simulink model "dx_hand_model"  (R2017b)
settings: Solver=ode3  StartTime=0.0  StopTime=inf  FixedStep=0.01  RelTol=1e-3  EnableMultiTasking=on
InitFcn:
  | cutFreq = 0.1; % T
  | sampleTime = 0.01;
  | filt = tf(1,[cutFreq 1]);
  | filt = c2d(filt,sampleTime);
  | 
  | cutFreq2 = 1;
  | filt2 = tf(1,[cutFreq2 1]);
  | filt2 = c2d(filt2,sampleTime);
  | 
  | cutFreq3 = 0.3;
  | filt3 = tf(1,[cutFreq3 1]);
  | filt3 = c2d(filt3,sampleTime);
  | 
  | update_param = 2;
  | 
  | ampliFactor = 1.60;
  | ampliFactorMiddle = 2.00;
  | ampliFactorDistal = 1;
  | 
  | % Set Hand Address
  | % RightHandAddress = '10.100.39.144';
  | RightHandAddress = '10.24.4.91';
  | Verosim = '10.100.39.22'
  | LeftHandAddress = '10.100.39.22'
  | 
  | max_force = 24; % Newton
model workspace (MAT data in the model file):
  SL_ROS_VariableLengthArrays_MaxSizes : struct (value not decoded)
libraries: robotlib x136, simulink_extras x27, simulink x16, etargetslib x2, dspnetwork x2
(part 9 of 19)

== matlab function dx_hand_model/Thumb/Direct Kinematics/get H/MATLAB Function3 ==
  data: xI input; xH_sol output; yI input; zI input; xJ input; yJ input; zJ input; xD input; yD input; zD input; yH_sol output; zH_sol output; xold input; yold input; zold input
function [xH_sol,yH_sol,zH_sol] = findH_optimized(xI,yI,zI,xJ,yJ,zJ,xD,yD,zD,xold,yold,zold)
%FINDH_OPTIMIZED
%    [XH_SOL,YH_SOL,ZH_SOL] = FINDH_OPTIMIZED(XD,XI,XJ,YD,YI,YJ,ZD,ZI,ZJ)

%    This function was generated by the Symbolic Math Toolbox version 8.0.
%    08-Feb-2018 20:19:06

t2 = xD.^2;
t3 = xI.^2;
t4 = yD.^2;
t5 = yI.^2;
t6 = zD.^2;
t7 = zI.^2;
t8 = xD.*yI;
t9 = xJ.*yD;
t10 = xI.*yJ;
t645 = xI.*yD;
t646 = xD.*yJ;
t647 = xJ.*yI;
t11 = t8+t9+t10-t645-t646-t647;
t12 = 1.0./t11;
t13 = yJ.^2;
t14 = xJ.^2;
t15 = zJ.^2;
t16 = t3.^2;
t17 = t5.^2;
t88 = t2.*t7.*zI.*8.0;
t89 = t3.*t6.*zD.*4.0;
t90 = t6.*t14.*zD.*4.0;
t91 = t7.*t14.*zI.*4.0;
t92 = t4.*t7.*zI.*8.0;
t93 = t5.*t6.*zD.*4.0;
t94 = t6.*t13.*zD.*4.0;
t95 = t7.*t13.*zI.*4.0;
t96 = t3.*zD.*1.4916e4;
t97 = t16.*zD.*4.0;
t98 = t14.*zD.*1.4916e4;
t99 = t3.*zJ.*1.4916e4;
t100 = t14.*zI.*1.4916e4;
t101 = t16.*zJ.*4.0;
t102 = t5.*zD.*1.4916e4;
t103 = t17.*zD.*4.0;
t104 = t13.*zD.*1.4916e4;
t105 = t5.*zJ.*1.4916e4;
t106 = t13.*zI.*1.4916e4;
t107 = t17.*zJ.*4.0;
t108 = t3.*xD.*xI.*zD.*8.0;
t109 = t7.*xD.*xI.*zI.*4.0;
t110 = t3.*xD.*xI.*zI.*4.0;
t111 = t2.*xD.*xI.*zI.*4.0;
t112 = t7.*xD.*xJ.*zI.*1.2e1;
t113 = t3.*xD.*xI.*zJ.*1.2e1;
t114 = t6.*xI.*xJ.*zD.*8.0;
t115 = t2.*xD.*xI.*zJ.*4.0;
t116 = t2.*xD.*xJ.*zI.*4.0;
t117 = t3.*xI.*xJ.*zD.*8.0;
t118 = t2.*xD.*xJ.*zJ.*4.0;
t119 = t7.*xI.*xJ.*zI.*4.0;
t120 = t3.*xI.*xJ.*zI.*4.0;
t121 = t3.*xI.*xJ.*zJ.*4.0;
t122 = t5.*yD.*yI.*zD.*8.0;
t123 = t7.*yD.*yI.*zI.*4.0;
t124 = t5.*yD.*yI.*zI.*4.0;
t125 = t4.*yD.*yI.*zI.*4.0;
t126 = t7.*yD.*yJ.*zI.*1.2e1;
t127 = t5.*yD.*yI.*zJ.*1.2e1;
t128 = t6.*yI.*yJ.*zD.*8.0;
t129 = t4.*yD.*yI.*zJ.*4.0;
t130 = t4.*yD.*yJ.*zI.*4.0;
t131 = t5.*yI.*yJ.*zD.*8.0;
t132 = t4.*yD.*yJ.*zJ.*4.0;
t133 = t7.*yI.*yJ.*zI.*4.0;
t134 = t5.*yI.*yJ.*zI.*4.0;
t135 = t5.*yI.*yJ.*zJ.*4.0;
t136 = t2.*t3.*zD.*4.0;
t137 = t2.*t14.*zD.*4.0;
t138 = t2.*t3.*zI.*8.0;
t139 = t2.*t3.*zJ.*1.2e1;
t140 = t2.*t14.*zI.*4.0;
t141 = t3.*t14.*zD.*4.0;
t142 = t3.*t14.*zI.*4.0;
t143 = t2.*t5.*zD.*4.0;
t144 = t3.*t4.*zD.*4.0;
t145 = t2.*t13.*zD.*4.0;
t146 = t4.*t14.*zD.*4.0;
t147 = t2.*t5.*zI.*8.0;
t148 = t3.*t4.*zI.*8.0;
t149 = t3.*t5.*zD.*8.0;
t150 = t2.*t5.*zJ.*4.0;
t151 = t2.*t13.*zI.*4.0;
t152 = t3.*t4.*zJ.*4.0;
t153 = t3.*t13.*zD.*4.0;
t154 = t4.*t14.*zI.*4.0;
t155 = t5.*t14.*zD.*4.0;
t156 = t3.*t5.*zJ.*8.0;
t157 = t3.*t13.*zI.*4.0;
t158 = t5.*t14.*zI.*4.0;
t159 = t4.*t5.*zD.*4.0;
t160 = t4.*t13.*zD.*4.0;
t161 = t3.*t7.*zD.*4.0;
t162 = t4.*t5.*zI.*8.0;
t163 = t2.*t15.*zI.*8.0;
t164 = t2.*t7.*zJ.*1.6e1;
t165 = t3.*t6.*zJ.*4.0;
t166 = t7.*t14.*zD.*4.0;
t167 = t6.*t14.*zI.*4.0;
t168 = t4.*t5.*zJ.*1.2e1;
t169 = t4.*t13.*zI.*4.0;
t170 = t5.*t13.*zD.*4.0;
t171 = t3.*t15.*zI.*8.0;
t172 = t3.*t7.*zJ.*4.0;
t173 = t5.*t13.*zI.*4.0;
t174 = t5.*t7.*zD.*4.0;
t175 = t4.*t15.*zI.*8.0;
t176 = t4.*t7.*zJ.*1.6e1;
t177 = t5.*t6.*zJ.*4.0;
t178 = t7.*t13.*zD.*4.0;
t179 = t6.*t13.*zI.*4.0;
t180 = t5.*t15.*zI.*8.0;
t181 = t5.*t7.*zJ.*4.0;
t182 = xD.*xI.*zI.*1.4916e4;
t183 = xD.*xI.*zJ.*1.4916e4;
t184 = xD.*xJ.*zI.*1.4916e4;
t185 = xI.*xJ.*zD.*2.9832e4;
t186 = xD.*xJ.*zJ.*1.4916e4;
t187 = xI.*xJ.*zI.*1.4916e4;
t188 = xI.*xJ.*zJ.*1.4916e4;
t189 = yD.*yI.*zI.*1.4916e4;
t190 = yD.*yI.*zJ.*1.4916e4;
t191 = yD.*yJ.*zI.*1.4916e4;
t192 = yI.*yJ.*zD.*2.9832e4;
t193 = yD.*yJ.*zJ.*1.4916e4;
t194 = yI.*yJ.*zI.*1.4916e4;
t195 = yI.*yJ.*zJ.*1.4916e4;
t196 = t14.*xD.*xI.*zD.*8.0;
t197 = t3.*xD.*xJ.*zD.*1.6e1;
t198 = t2.*xI.*xJ.*zD.*8.0;
t199 = t14.*xD.*xI.*zI.*8.0;
t200 = t3.*xD.*xJ.*zI.*4.0;
t201 = t2.*xI.*xJ.*zI.*4.0;
t202 = t3.*xD.*xJ.*zJ.*1.2e1;
t203 = t2.*xI.*xJ.*zJ.*1.2e1;
t204 = t4.*xD.*xI.*zI.*4.0;
t205 = t5.*xD.*xI.*zD.*8.0;
t206 = t4.*xD.*xI.*zJ.*4.0;
t207 = t13.*xD.*xI.*zD.*8.0;
t208 = t4.*xD.*xJ.*zI.*4.0;
t209 = t4.*xI.*xJ.*zD.*8.0;
t210 = t4.*xD.*xJ.*zJ.*4.0;
t211 = t5.*xD.*xI.*zI.*4.0;
t212 = t5.*xD.*xI.*zJ.*1.2e1;
t213 = t13.*xD.*xI.*zI.*8.0;
t214 = t5.*xD.*xJ.*zI.*1.2e1;
t215 = t4.*xI.*xJ.*zI.*1.2e1;
t216 = t5.*xI.*xJ.*zD.*8.0;
t217 = t5.*xD.*xJ.*zJ.*4.0;
t218 = t4.*xI.*xJ.*zJ.*4.0;
t219 = t5.*xI.*xJ.*zI.*4.0;
t220 = t5.*xI.*xJ.*zJ.*4.0;
t221 = t7.*xD.*xI.*zD.*8.0;
t222 = t6.*xD.*xI.*zI.*4.0;
t223 = t2.*yD.*yI.*zI.*4.0;
t224 = t3.*yD.*yI.*zD.*8.0;
t225 = t6.*xD.*xI.*zJ.*4.0;
t226 = t7.*xD.*xJ.*zD.*8.0;
t227 = t6.*xD.*xJ.*zI.*4.0;
t228 = t2.*yD.*yI.*zJ.*4.0;
t229 = t2.*yD.*yJ.*zI.*4.0;
t230 = t2.*yI.*yJ.*zD.*8.0;
t231 = t14.*yD.*yI.*zD.*8.0;
t232 = t6.*xD.*xJ.*zJ.*4.0;
t233 = t2.*yD.*yJ.*zJ.*4.0;
t234 = t3.*yD.*yI.*zI.*4.0;
t235 = t15.*xD.*xI.*zI.*1.6e1;
t236 = t7.*xD.*xI.*zJ.*2.0e1;
t237 = t6.*xI.*xJ.*zI.*4.0;
t238 = t2.*yI.*yJ.*zI.*1.2e1;
t239 = t3.*yD.*yI.*zJ.*1.2e1;
t240 = t3.*yD.*yJ.*zI.*1.2e1;
t241 = t3.*yI.*yJ.*zD.*8.0;
t242 = t14.*yD.*yI.*zI.*8.0;
t243 = t7.*xD.*xJ.*zJ.*1.2e1;
t244 = t6.*xI.*xJ.*zJ.*4.0;
t245 = t2.*yI.*yJ.*zJ.*4.0;
t246 = t3.*yD.*yJ.*zJ.*4.0;
t247 = t3.*yI.*yJ.*zI.*4.0;
t248 = t7.*xI.*xJ.*zJ.*1.2e1;
t249 = t3.*yI.*yJ.*zJ.*4.0;
t250 = t13.*yD.*yI.*zD.*8.0;
t251 = t5.*yD.*yJ.*zD.*1.6e1;
t252 = t4.*yI.*yJ.*zD.*8.0;
t253 = t13.*yD.*yI.*zI.*8.0;
t254 = t5.*yD.*yJ.*zI.*4.0;
t255 = t4.*yI.*yJ.*zI.*4.0;
t256 = t5.*yD.*yJ.*zJ.*1.2e1;
t257 = t4.*yI.*yJ.*zJ.*1.2e1;
t258 = t7.*yD.*yI.*zD.*8.0;
t259 = t6.*yD.*yI.*zI.*4.0;
t260 = t6.*yD.*yI.*zJ.*4.0;
t261 = t7.*yD.*yJ.*zD.*8.0;
t262 = t6.*yD.*yJ.*zI.*4.0;
t263 = t6.*yD.*yJ.*zJ.*4.0;
t264 = t15.*yD.*yI.*zI.*1.6e1;
t265 = t7.*yD.*yI.*zJ.*2.0e1;
t266 = t6.*yI.*yJ.*zI.*4.0;
t267 = t3.*zD.*zI.*zJ.*8.0;
t268 = t7.*yD.*yJ.*zJ.*1.2e1;
t269 = t6.*yI.*yJ.*zJ.*4.0;
t270 = t7.*yI.*yJ.*zJ.*1.2e1;
t271 = t5.*zD.*zI.*zJ.*8.0;
t272 = xD.*xI.*yD.*yI.*zJ.*1.6e1;
t273 = xD.*xI.*yD.*yJ.*zI.*8.0;
t274 = xD.*xI.*yI.*yJ.*zD.*1.6e1;
t275 = xD.*xJ.*yD.*yI.*zI.*8.0;
t276 = xI.*xJ.*yD.*yI.*zD.*1.6e1;
t277 = xD.*xI.*yD.*yJ.*zJ.*8.0;
t278 = xD.*xJ.*yD.*yI.*zJ.*8.0;
t279 = xD.*xJ.*yD.*yJ.*zI.*1.6e1;
t280 = xD.*xI.*yI.*yJ.*zI.*8.0;
t281 = xI.*xJ.*yD.*yI.*zI.*8.0;
t282 = xD.*xI.*yI.*yJ.*zJ.*8.0;
t283 = xD.*xJ.*yI.*yJ.*zI.*1.6e1;
t284 = xI.*xJ.*yD.*yI.*zJ.*8.0;
t285 = xI.*xJ.*yD.*yJ.*zI.*1.6e1;
t286 = xI.*xJ.*yI.*yJ.*zI.*1.6e1;
t287 = xD.*xI.*zD.*zI.*zJ.*8.0;
t288 = xD.*xJ.*zD.*zI.*zJ.*8.0;
t289 = xI.*xJ.*zD.*zI.*zJ.*8.0;
t290 = yD.*yI.*zD.*zI.*zJ.*8.0;
t291 = yD.*yJ.*zD.*zI.*zJ.*8.0;
t292 = yI.*yJ.*zD.*zI.*zJ.*8.0;
t18 = t88+t89+t90+t91+t92+t93+t94+t95-t96+t97-t98+t99+t100-t101-t102+t103-t104+t105+t106-t107-t108-t109-t110-t111-t112+t113-t114+t115+t116-t117-t118+t119+t120+t121-t122-t123-t124-t125-t126+t127-t128+t129+t130-t131-t132+t133+t134+t135+t136+t137+t138-t139-t140+t141-t142+t143+t144+t145+t146+t147+t148+t149-t150+t151-t152+t153+t154+t155-t156+t157+t158+t159+t160+t161+t162+t163-t164-t165-t166-t167-t168-t169+t170+t171-t172-t173+t174+t175-t176-t177-t178-t179+t180-t181+t182-t183-t184+t185+t186-t187-t188+t189-t190-t191+t192+t193-t194-t195-t196+t197-t198+t199-t200-t201-t202+t203-t204-t205+t206-t207+t208-t209-t210-t211+t212-t213-t214-t215-t216-t217+t218+t219+t220-t221-t222-t223-t224+t225+t226+t227+t228+t229-t230-t231-t232-t233-t234-t235+t236+t237-t238+t239-t240-t241-t242+t243+t244+t245-t246+t247-t248+t249-t250+t251-t252+t253-t254-t255-t256+t257-t258-t259+t260+t261+t262-t263-t264+t265+t266-t267+t268+t269-t270-t271-t272+t273+t274+t275+t276+t277+t278-t279+t280+t281-t282+t283-t284+t285-t286+t287-t288+t289+t290-t291+t292;
t19 = t2.*t5.*4.0;
t20 = t3.*t4.*4.0;
t21 = t2.*t13.*4.0;
t22 = t4.*t14.*4.0;
t23 = t3.*t13.*4.0;
t24 = t5.*t14.*4.0;
t25 = t2.*t7.*4.0;
t26 = t3.*t6.*4.0;
t27 = t2.*t15.*4.0;
t28 = t6.*t14.*4.0;
t29 = t3.*t15.*4.0;
t30 = t7.*t14.*4.0;
t31 = t4.*t7.*4.0;
t32 = t5.*t6.*4.0;
t33 = t4.*t15.*4.0;
t34 = t6.*t13.*4.0;
t35 = t5.*t15.*4.0;
t36 = t7.*t13.*4.0;
t37 = xD.*xI.*yD.*yJ.*8.0;
t38 = xD.*xJ.*yD.*yI.*8.0;
t39 = xD.*xI.*yI.*yJ.*8.0;
t40 = xI.*xJ.*yD.*yI.*8.0;
t41 = xD.*xJ.*yI.*yJ.*8.0;
t42 = xI.*xJ.*yD.*yJ.*8.0;
t43 = xD.*xI.*zD.*zJ.*8.0;
t44 = xD.*xJ.*zD.*zI.*8.0;
t45 = xD.*xI.*zI.*zJ.*8.0;
t46 = xI.*xJ.*zD.*zI.*8.0;
t47 = xD.*xJ.*zI.*zJ.*8.0;
t48 = xI.*xJ.*zD.*zJ.*8.0;
t49 = yD.*yI.*zD.*zJ.*8.0;
t50 = yD.*yJ.*zD.*zI.*8.0;
t51 = yD.*yI.*zI.*zJ.*8.0;
t52 = yI.*yJ.*zD.*zI.*8.0;
t53 = yD.*yJ.*zI.*zJ.*8.0;
t54 = yI.*yJ.*zD.*zJ.*8.0;
t60 = t13.*xD.*xI.*8.0;
t61 = t5.*xD.*xJ.*8.0;
t62 = t4.*xI.*xJ.*8.0;
t63 = t15.*xD.*xI.*8.0;
t64 = t7.*xD.*xJ.*8.0;
t65 = t6.*xI.*xJ.*8.0;
t66 = t2.*yI.*yJ.*8.0;
t67 = t3.*yD.*yJ.*8.0;
t68 = t14.*yD.*yI.*8.0;
t69 = t15.*yD.*yI.*8.0;
t70 = t7.*yD.*yJ.*8.0;
t71 = t6.*yI.*yJ.*8.0;
t72 = t2.*zI.*zJ.*8.0;
t73 = t3.*zD.*zJ.*8.0;
t74 = t14.*zD.*zI.*8.0;
t75 = t4.*zI.*zJ.*8.0;
t76 = t5.*zD.*zJ.*8.0;
t77 = t13.*zD.*zI.*8.0;
t78 = xD.*xI.*yD.*yI.*8.0;
t79 = xD.*xJ.*yD.*yJ.*8.0;
t80 = xI.*xJ.*yI.*yJ.*8.0;
t81 = xD.*xI.*zD.*zI.*8.0;
t82 = xD.*xJ.*zD.*zJ.*8.0;
t83 = xI.*xJ.*zI.*zJ.*8.0;
t84 = yD.*yI.*zD.*zI.*8.0;
t85 = yD.*yJ.*zD.*zJ.*8.0;
t86 = yI.*yJ.*zI.*zJ.*8.0;
t55 = t19+t20+t21+t22+t23+t24+t25+t26+t27+t28+t29+t30+t31+t32+t33+t34+t35+t36+t37+t38+t39+t40+t41+t42+t43+t44+t45+t46+t47+t48+t49+t50+t51+t52+t53+t54-t60-t61-t62-t63-t64-t65-t66-t67-t68-t69-t70-t71-t72-t73-t74-t75-t76-t77-t78-t79-t80-t81-t82-t83-t84-t85-t86;
t56 = t2.^2;
t57 = t4.^2;
t58 = t6.^2;
t59 = t7.^2;
t87 = 1.0./t55.^2;
t293 = t18.^2;
t294 = t87.*t293.*(1.0./4.0);
t295 = 1.0./t55;
t296 = t2.*t16.*6.0;
t297 = t3.*t56;
t298 = t14.*t56;
t299 = t14.*t16;
t300 = t2.*t17.*2.0;
t301 = t5.*t56;
t302 = t3.*t57;
t303 = t4.*t16.*2.0;
t304 = t13.*t56;
t305 = t14.*t57;
t306 = t3.*t17.*3.0;
t307 = t5.*t16.*3.0;
t308 = t13.*t16;
t309 = t14.*t17;
t310 = t2.*t59.*4.0;
t311 = t3.*t58;
t312 = t6.*t16.*2.0;
t313 = t4.*t17.*6.0;
t314 = t5.*t57;
t315 = t14.*t58;
t316 = t13.*t57;
t317 = t3.*t59;
t318 = t7.*t16.*2.0;
t319 = t7.*t14.*7.458e3;
t320 = t14.*t59;
t321 = t13.*t17;
t322 = t4.*t59.*4.0;
t323 = t5.*t58;
t324 = t6.*t17.*2.0;
t325 = t13.*t58;
t326 = t5.*t59;
t327 = t7.*t17.*2.0;
t328 = t7.*t13.*7.458e3;
t329 = t13.*t59;
t330 = t3.*xD.*xI.*1.4916e4;
t331 = t3.*xI.*xJ.*1.4916e4;
t332 = t5.*yD.*yI.*1.4916e4;
t333 = t5.*yI.*yJ.*1.4916e4;
t334 = t3.*1.3905441e7;
t335 = t14.*1.3905441e7;
t336 = t5.*1.3905441e7;
t337 = t13.*1.3905441e7;
t338 = t14.*xD.*xI.*1.4916e4;
t339 = t2.*xI.*xJ.*1.4916e4;
t340 = t16.*xD.*xJ.*8.0;
t341 = t5.*xD.*xI.*1.4916e4;
t342 = t13.*xD.*xI.*2.7716e4;
t343 = t5.*xD.*xJ.*1.28e4;
t344 = t4.*xI.*xJ.*2.7716e4;
t345 = t5.*xI.*xJ.*1.4916e4;
t346 = t7.*xD.*xI.*1.4916e4;
t347 = t3.*yD.*yI.*1.4916e4;
t348 = t6.*xI.*xJ.*1.4916e4;
t349 = t2.*yI.*yJ.*2.7716e4;
t350 = t3.*yD.*yJ.*1.28e4;
t351 = t14.*yD.*yI.*2.7716e4;
t352 = t3.*yI.*yJ.*1.4916e4;
t353 = t59.*xI.*xJ.*2.0;
t354 = t13.*yD.*yI.*1.4916e4;
t355 = t4.*yI.*yJ.*1.4916e4;
t356 = t17.*yD.*yJ.*8.0;
t357 = t7.*yD.*yI.*1.4916e4;
t358 = t6.*yI.*yJ.*1.4916e4;
t359 = t3.*zI.*zJ.*1.4916e4;
t360 = t59.*yI.*yJ.*2.0;
t361 = t5.*zI.*zJ.*1.4916e4;
t362 = t2.*t3.*xD.*xJ.*8.0;
t363 = t2.*t7.*xD.*xJ.*4.0;
t364 = t4.*t5.*yD.*yJ.*8.0;
t365 = t4.*t7.*yD.*yJ.*4.0;
t366 = t2.*t3.*t14.*6.0;
t367 = t2.*t3.*t4.*2.0;
t368 = t2.*t4.*t14.*2.0;
t369 = t2.*t3.*t5.*8.0;
t370 = t2.*t3.*t13.*6.0;
t371 = t2.*t5.*t14.*2.0;
t372 = t3.*t4.*t14.*2.0;
t373 = t3.*t5.*t14.*2.0;
t374 = t2.*t3.*t6.*2.0;
t375 = t2.*t4.*t5.*2.0;
t376 = t2.*t6.*t14.*2.0;
t377 = t2.*t4.*t13.*2.0;
t378 = t2.*t3.*t7.*1.0e1;
t379 = t3.*t4.*t5.*8.0;
t380 = t2.*t5.*t13.*2.0;
t381 = t3.*t6.*t14.*2.0;
t382 = t3.*t4.*t13.*2.0;
t383 = t4.*t5.*t14.*6.0;
t384 = t3.*t5.*t13.*2.0;
t385 = t2.*t5.*t6.*2.0;
t386 = t3.*t4.*t6.*2.0;
t387 = t2.*t6.*t13.*2.0;
t388 = t4.*t6.*t14.*2.0;
t389 = t2.*t5.*t7.*6.0;
t390 = t3.*t4.*t7.*6.0;
t391 = t3.*t5.*t6.*4.0;
t392 = t2.*t7.*t13.*2.0;
t393 = t3.*t6.*t13.*2.0;
t394 = t4.*t7.*t14.*2.0;
t395 = t5.*t6.*t14.*2.0;
t396 = t4.*t5.*t13.*6.0;
t397 = t3.*t5.*t7.*4.0;
t398 = t3.*t7.*t13.*2.0;
t399 = t5.*t7.*t14.*2.0;
t400 = t4.*t5.*t6.*2.0;
t401 = t4.*t6.*t13.*2.0;
t402 = t3.*t6.*t7.*2.0;
t403 = t4.*t5.*t7.*1.0e1;
t404 = t2.*t7.*t15.*4.0;
t405 = t5.*t6.*t13.*2.0;
t406 = t3.*t7.*t15.*4.0;
t407 = t5.*t6.*t7.*2.0;
t408 = t4.*t7.*t15.*4.0;
t409 = t5.*t7.*t15.*4.0;
t410 = t3.*t4.*xD.*xJ.*8.0;
t411 = t3.*t5.*xD.*xJ.*8.0;
t412 = t3.*t6.*xD.*xJ.*8.0;
t413 = t7.*t14.*xD.*xI.*4.0;
t414 = t3.*t7.*xD.*xJ.*4.0;
t415 = t4.*t7.*xD.*xJ.*4.0;
t416 = t2.*t5.*yD.*yJ.*8.0;
t417 = t3.*t5.*yD.*yJ.*8.0;
t418 = t6.*t7.*xD.*xJ.*4.0;
t419 = t2.*t7.*yD.*yJ.*4.0;
t420 = t5.*t6.*yD.*yJ.*8.0;
t421 = t7.*t13.*yD.*yI.*4.0;
t422 = t5.*t7.*yD.*yJ.*4.0;
t423 = t6.*t7.*yD.*yJ.*4.0;
t424 = xD.*xI.*yD.*yI.*1.28e4;
t425 = xD.*xJ.*yD.*yJ.*1.28e4;
t426 = xI.*xJ.*yI.*yJ.*1.28e4;
t427 = xD.*xJ.*zI.*zJ.*1.4916e4;
t428 = yD.*yJ.*zI.*zJ.*1.4916e4;
t429 = t5.*xD.*xI.*yD.*yI.*8.0;
t430 = t3.*xD.*xI.*yD.*yI.*8.0;
t431 = t5.*xD.*xI.*yI.*yJ.*8.0;
t432 = t3.*xD.*xI.*yI.*yJ.*8.0;
t433 = t5.*xI.*xJ.*yD.*yI.*8.0;
t434 = t4.*xI.*xJ.*yD.*yI.*8.0;
t435 = t2.*xD.*xI.*yI.*yJ.*8.0;
t436 = t3.*xI.*xJ.*yD.*yI.*8.0;
t437 = t7.*xD.*xI.*zI.*zJ.*1.2e1;
t438 = t3.*xD.*xI.*zI.*zJ.*1.2e1;
t439 = t2.*xD.*xI.*zI.*zJ.*4.0;
t440 = t7.*xD.*xJ.*zI.*zJ.*4.0;
t441 = t3.*xI.*xJ.*zI.*zJ.*4.0;
t442 = t7.*yD.*yI.*zI.*zJ.*1.2e1;
t443 = t5.*yD.*yI.*zI.*zJ.*1.2e1;
t444 = t4.*yD.*yI.*zI.*zJ.*4.0;
t445 = t7.*yD.*yJ.*zI.*zJ.*4.0;
t446 = t5.*yI.*yJ.*zI.*zJ.*4.0;
t447 = t14.*xD.*xI.*yD.*yI.*8.0;
t448 = t2.*xI.*xJ.*yD.*yI.*8.0;
t449 = t13.*xD.*xI.*yD.*yI.*8.0;
t450 = t4.*xD.*xI.*yI.*yJ.*8.0;
t451 = t7.*xD.*xI.*yD.*yI.*8.0;
t452 = t6.*xD.*xI.*yI.*yJ.*8.0;
t453 = t6.*xI.*xJ.*yD.*yI.*8.0;
t454 = t7.*xD.*xI.*yI.*yJ.*8.0;
t455 = t7.*xI.*xJ.*yD.*yI.*8.0;
t456 = t7.*xD.*xJ.*yI.*yJ.*8.0;
t457 = t7.*xI.*xJ.*yD.*yJ.*8.0;
t458 = t2.*xI.*xJ.*zI.*zJ.*1.2e1;
t459 = t4.*xD.*xI.*zI.*zJ.*4.0;
t460 = t5.*xD.*xI.*zI.*zJ.*1.2e1;
t461 = t4.*xI.*xJ.*zI.*zJ.*4.0;
t462 = t5.*xI.*xJ.*zI.*zJ.*4.0;
t463 = t6.*xD.*xI.*zI.*zJ.*4.0;
t464 = t2.*yD.*yI.*zI.*zJ.*4.0;
t465 = t3.*yD.*yI.*zI.*zJ.*1.2e1;
t466 = t6.*xI.*xJ.*zI.*zJ.*4.0;
t467 = t2.*yI.*yJ.*zI.*zJ.*4.0;
t468 = t3.*yI.*yJ.*zI.*zJ.*4.0;
t469 = t4.*yI.*yJ.*zI.*zJ.*1.2e1;
t470 = t6.*yD.*yI.*zI.*zJ.*4.0;
t471 = t6.*yI.*yJ.*zI.*zJ.*4.0;
t472 = xD.*xI.*yD.*yJ.*zI.*zJ.*8.0;
t473 = xD.*xJ.*yD.*yI.*zI.*zJ.*8.0;
t477 = t2.*t3.*7.458e3;
t478 = t2.*t3.*xD.*xI.*4.0;
t479 = t2.*t14.*7.458e3;
t480 = t3.*t14.*7.458e3;
t481 = t2.*t5.*1.3858e4;
t482 = t3.*t4.*1.3858e4;
t483 = t2.*t13.*1.3858e4;
t484 = t4.*t14.*1.3858e4;
t485 = t3.*t5.*1.4916e4;
t486 = t3.*t13.*1.3858e4;
t487 = t5.*t14.*1.3858e4;
t488 = t3.*t6.*7.458e3;
t489 = t4.*t5.*7.458e3;
t490 = t4.*t5.*yD.*yI.*4.0;
t491 = t6.*t14.*7.458e3;
t492 = t4.*t13.*7.458e3;
t493 = t3.*t7.*7.458e3;
t494 = t5.*t13.*7.458e3;
t495 = t5.*t6.*7.458e3;
t496 = t6.*t13.*7.458e3;
t497 = t5.*t7.*7.458e3;
t498 = xI.*xJ.*2.7810882e7;
t499 = yI.*yJ.*2.7810882e7;
t500 = t16.*xD.*xI.*4.0;
t501 = t16.*xI.*xJ.*2.0;
t502 = t17.*yD.*yI.*4.0;
t503 = t17.*yI.*yJ.*2.0;
t504 = t16.*7.458e3;
t505 = t17.*7.458e3;
t506 = t3.*xD.*xJ.*2.9832e4;
t507 = t56.*xI.*xJ.*2.0;
t508 = t17.*xD.*xI.*4.0;
t509 = t57.*xI.*xJ.*2.0;
t510 = t17.*xI.*xJ.*2.0;
t511 = t59.*xD.*xI.*4.0;
t512 = t16.*yD.*yI.*4.0;
t513 = t7.*xD.*xJ.*1.4916e4;
t514 = t59.*xD.*xJ.*4.0;
t515 = t58.*xI.*xJ.*2.0;
t516 = t56.*yI.*yJ.*2.0;
t517 = t16.*yI.*yJ.*2.0;
t518 = t5.*yD.*yJ.*2.9832e4;
t519 = t57.*yI.*yJ.*2.0;
t520 = t59.*yD.*yI.*4.0;
t521 = t7.*yD.*yJ.*1.4916e4;
t522 = t59.*yD.*yJ.*4.0;
t523 = t58.*yI.*yJ.*2.0;
t524 = t16.*zI.*zJ.*4.0;
t525 = t17.*zI.*zJ.*4.0;
t526 = t3.*t14.*xD.*xI.*4.0;
t527 = t2.*t3.*xI.*xJ.*1.2e1;
t528 = t2.*t14.*xD.*xI.*4.0;
t529 = t3.*t4.*xD.*xI.*4.0;
t530 = t3.*t5.*xD.*xI.*8.0;
t531 = t2.*t5.*xD.*xI.*4.0;
t532 = t3.*t13.*xD.*xI.*4.0;
t533 = t2.*t13.*xD.*xI.*4.0;
t534 = t3.*t4.*xI.*xJ.*4.0;
t535 = t3.*t5.*xI.*xJ.*4.0;
t536 = t3.*t6.*xD.*xI.*4.0;
t537 = t2.*t5.*yD.*yI.*4.0;
t538 = t3.*t7.*xD.*xI.*8.0;
t539 = t2.*t7.*xD.*xI.*4.0;
t540 = t3.*t5.*yD.*yI.*8.0;
t541 = t3.*t4.*yD.*yI.*4.0;
t542 = t2.*t5.*yI.*yJ.*4.0;
t543 = t3.*t6.*xI.*xJ.*4.0;
t544 = t5.*t14.*yD.*yI.*4.0;
t545 = t4.*t14.*yD.*yI.*4.0;
t546 = t3.*t5.*yI.*yJ.*4.0;
t547 = t5.*t13.*yD.*yI.*4.0;
t548 = t4.*t5.*yI.*yJ.*1.2e1;
t549 = t4.*t13.*yD.*yI.*4.0;
t550 = t5.*t6.*yD.*yI.*4.0;
t551 = t5.*t7.*yD.*yI.*8.0;
t552 = t4.*t7.*yD.*yI.*4.0;
t553 = t2.*t7.*zI.*zJ.*8.0;
t554 = t5.*t6.*yI.*yJ.*4.0;
t555 = t3.*t7.*zI.*zJ.*4.0;
t556 = t4.*t7.*zI.*zJ.*8.0;
t557 = t5.*t7.*zI.*zJ.*4.0;
t558 = t2.*t7.*t14.*2.0;
t559 = t3.*t7.*t14.*2.0;
t560 = t6.*t7.*t14.*2.0;
t561 = t4.*t7.*t13.*2.0;
t562 = t5.*t7.*t13.*2.0;
t563 = t6.*t7.*t13.*2.0;
t564 = t4.*t14.*xD.*xI.*4.0;
t565 = t2.*t4.*xI.*xJ.*4.0;
t566 = t5.*t14.*xD.*xI.*4.0;
t567 = t2.*t5.*xI.*xJ.*4.0;
t568 = t4.*t5.*xD.*xI.*4.0;
t569 = t2.*t3.*yD.*yI.*4.0;
t570 = t6.*t14.*xD.*xI.*4.0;
t571 = t4.*t13.*xD.*xI.*4.0;
t572 = t2.*t6.*xI.*xJ.*4.0;
t573 = t2.*t14.*yD.*yI.*4.0;
t574 = t5.*t13.*xD.*xI.*4.0;
t575 = t4.*t5.*xI.*xJ.*1.2e1;
t576 = t2.*t7.*xI.*xJ.*8.0;
t577 = t2.*t3.*yI.*yJ.*1.2e1;
t578 = t3.*t14.*yD.*yI.*4.0;
t579 = t4.*t7.*xD.*xI.*4.0;
t580 = t5.*t6.*xD.*xI.*4.0;
t581 = t6.*t13.*xD.*xI.*4.0;
t582 = t4.*t6.*xI.*xJ.*4.0;
t583 = t2.*t13.*yD.*yI.*4.0;
t584 = t2.*t4.*yI.*yJ.*4.0;
t585 = t5.*t7.*xD.*xI.*8.0;
t586 = t7.*t13.*xD.*xI.*4.0;
t587 = t5.*t7.*xD.*xJ.*4.0;
t588 = t4.*t7.*xI.*xJ.*8.0;
t589 = t5.*t6.*xI.*xJ.*4.0;
t590 = t3.*t13.*yD.*yI.*4.0;
t591 = t3.*t4.*yI.*yJ.*4.0;
t592 = t6.*t7.*xD.*xI.*4.0;
t593 = t2.*t7.*yD.*yI.*4.0;
t594 = t3.*t6.*yD.*yI.*4.0;
t595 = t2.*t6.*yI.*yJ.*4.0;
t596 = t6.*t14.*yD.*yI.*4.0;
t597 = t3.*t7.*yD.*yI.*8.0;
t598 = t7.*t15.*xD.*xI.*8.0;
t599 = t2.*t7.*yI.*yJ.*8.0;
t600 = t2.*t3.*zI.*zJ.*1.2e1;
t601 = t3.*t7.*yD.*yJ.*4.0;
t602 = t3.*t6.*yI.*yJ.*4.0;
t603 = t7.*t14.*yD.*yI.*4.0;
t604 = t6.*t13.*yD.*yI.*4.0;
t605 = t4.*t6.*yI.*yJ.*4.0;
t606 = t2.*t5.*zI.*zJ.*4.0;
t607 = t3.*t4.*zI.*zJ.*4.0;
t608 = t4.*t7.*yI.*yJ.*8.0;
t609 = t3.*t5.*zI.*zJ.*8.0;
t610 = t6.*t7.*yD.*yI.*4.0;
t611 = t7.*t15.*yD.*yI.*8.0;
t612 = t3.*t6.*zI.*zJ.*4.0;
t613 = t4.*t5.*zI.*zJ.*1.2e1;
t614 = t5.*t6.*zI.*zJ.*4.0;
t615 = xD.*xI.*yD.*yJ.*1.28e4;
t616 = xD.*xJ.*yD.*yI.*1.28e4;
t617 = xD.*xI.*yI.*yJ.*4.2632e4;
t618 = xI.*xJ.*yD.*yI.*4.2632e4;
t619 = xD.*xJ.*yI.*yJ.*1.28e4;
t620 = xI.*xJ.*yD.*yJ.*1.28e4;
t621 = xD.*xI.*zI.*zJ.*1.4916e4;
t622 = xI.*xJ.*zI.*zJ.*1.4916e4;
t623 = yD.*yI.*zI.*zJ.*1.4916e4;
t624 = yI.*yJ.*zI.*zJ.*1.4916e4;
t625 = t2.*xD.*xJ.*zI.*zJ.*4.0;
t626 = t7.*xI.*xJ.*zI.*zJ.*4.0;
t627 = t4.*yD.*yJ.*zI.*zJ.*4.0;
t628 = t7.*yI.*yJ.*zI.*zJ.*4.0;
t629 = t3.*xD.*xJ.*yD.*yI.*1.6e1;
t630 = t5.*xD.*xI.*yD.*yJ.*1.6e1;
t631 = t7.*xD.*xJ.*yD.*yJ.*8.0;
t632 = t3.*xD.*xJ.*zI.*zJ.*1.2e1;
t633 = t7.*xI.*xJ.*yI.*yJ.*8.0;
t634 = t4.*xD.*xJ.*zI.*zJ.*4.0;
t635 = t5.*xD.*xJ.*zI.*zJ.*4.0;
t636 = t6.*xD.*xJ.*zI.*zJ.*4.0;
t637 = t2.*yD.*yJ.*zI.*zJ.*4.0;
t638 = t3.*yD.*yJ.*zI.*zJ.*4.0;
t639 = t5.*yD.*yJ.*zI.*zJ.*1.2e1;
t640 = t6.*yD.*yJ.*zI.*zJ.*4.0;
t641 = xD.*xI.*yD.*yI.*zI.*zJ.*1.6e1;
t642 = xD.*xI.*yI.*yJ.*zI.*zJ.*8.0;
t643 = xI.*xJ.*yD.*yI.*zI.*zJ.*8.0;
t474 = t296+t297+t298+t299+t300+t301+t302+t303+t304+t305+t306+t307+t308+t309+t310+t311+t312+t313+t314+t315+t316+t317+t318+t319+t320+t321+t322+t323+t324+t325+t326+t327+t328+t329+t330+t331+t332+t333+t334+t335+t336+t337+t338+t339+t340+t341+t342+t343+t344+t345+t346+t347+t348+t349+t350+t351+t352+t353+t354+t355+t356+t357+t358+t359+t360+t361+t362+t363+t364+t365+t366+t367+t368+t369+t370+t371+t372+t373+t374+t375+t376+t377+t378+t379+t380+t381+t382+t383+t384+t385+t386+t387+t388+t389+t390+t391+t392+t393+t394+t395+t396+t397+t398+t399+t400+t401+t402+t403+t404+t405+t406+t407+t408+t409+t410+t411+t412+t413+t414+t415+t416+t417+t418+t419+t420+t421+t422+t423+t424+t425+t426+t427+t428+t429+t430+t431+t432+t433+t434+t435+t436+t437+t438+t439+t440+t441+t442+t443+t444+t445+t446+t447+t448+t449+t450+t451+t452+t453+t454+t455+t456+t457+t458+t459+t460+t461+t462+t463+t464+t465+t466+t467+t468+t469+t470+t471+t472+t473-t477-t478-t479-t480-t481-t482-t483-t484-t485-t486-t487-t488-t489-t490-t491-t492-t493-t494-t495-t496-t497-t498-t499-t500-t501-t502-t503-t504-t505-t506-t507-t508-t509-t510-t511-t512-t513-t514-t515-t516-t517-t518-t519-t520-t521-t522-t523-t524-t525-t526-t527-t528-t529-t530-t531-t532-t533-t534-t535-t536-t537-t538-t539-t540-t541-t542-t543-t544-t545-t546-t547-t548-t549-t550-t551-t552-t553-t554-t555-t556-t557-t558-t559-t560-t561-t562-t563-t564-t565-t566-t567-t568-t569-t570-t571-t572-t573-t574-t575-t576-t577-t578-t579-t580-t581-t582-t583-t584-t585-t586-t587-t588-t589-t590-t591-t592-t593-t594-t595-t596-t597-t598-t599-t600-t601-t602-t603-t604-t605-t606-t607-t608-t609-t610-t611-t612-t613-t614-t615-t616-t617-t618-t619-t620-t621-t622-t623-t624-t625-t626-t627-t628-t629-t630-t631-t632-t633-t634-t635-t636-t637-t638-t639-t640-t641-t642-t643+t3.*t16+t5.*t17;
t644 = t295.*t474;
t475 = t294-t644;
if (t475 < 0)
    xH_sol = complex(xold);
    yH_sol = complex(yold);
    zH_sol = complex(zold);
    %t475=single(0);
else
t476 = sqrt(complex(abs(t475)));
t648 = yJ.*3.729e3;
t649 = t2.*yI;
t650 = t3.*yI;
t651 = t3.*yJ;
t652 = t4.*yI;
t653 = t6.*yI;
t654 = t7.*yI;
t655 = t7.*yJ;
t656 = xI.*xJ.*yD.*2.0;
t657 = yD.*yI.*yJ.*2.0;
t658 = yD.*zI.*zJ.*2.0;
t659 = t648+t649+t650+t651+t652+t653+t654+t655+t656+t657+t658-yI.*3.729e3-t3.*yD.*2.0-t5.*yD.*2.0-t7.*yD.*2.0+t5.*yI-t2.*yJ-t4.*yJ-t5.*yJ-t6.*yJ-xI.*xJ.*yI.*2.0-yI.*zI.*zJ.*2.0;
t660 = t12.*t659.*(1.0./2.0);
t661 = yD.*zI;
t662 = yJ.*zD;
t663 = yI.*zJ;
t664 = t661+t662+t663-yI.*zD-yD.*zJ-yJ.*zI;
t665 = t2.*t5;
t666 = t3.*t4;
t667 = t2.*t13;
t668 = t4.*t14;
t669 = t3.*t13;
t670 = t5.*t14;
t671 = t2.*t7;
t672 = t3.*t6;
t673 = t2.*t15;
t674 = t6.*t14;
t675 = t3.*t15;
t676 = t7.*t14;
t677 = t4.*t7;
t678 = t5.*t6;
t679 = t4.*t15;
t680 = t6.*t13;
t681 = t5.*t15;
t682 = t7.*t13;
t683 = xD.*xI.*yD.*yJ.*2.0;
t684 = xD.*xJ.*yD.*yI.*2.0;
t685 = xD.*xI.*yI.*yJ.*2.0;
t686 = xI.*xJ.*yD.*yI.*2.0;
t687 = xD.*xJ.*yI.*yJ.*2.0;
t688 = xI.*xJ.*yD.*yJ.*2.0;
t689 = xD.*xI.*zD.*zJ.*2.0;
t690 = xD.*xJ.*zD.*zI.*2.0;
t691 = xD.*xI.*zI.*zJ.*2.0;
t692 = xI.*xJ.*zD.*zI.*2.0;
t693 = xD.*xJ.*zI.*zJ.*2.0;
t694 = xI.*xJ.*zD.*zJ.*2.0;
t695 = yD.*yI.*zD.*zJ.*2.0;
t696 = yD.*yJ.*zD.*zI.*2.0;
t697 = yD.*yI.*zI.*zJ.*2.0;
t698 = yI.*yJ.*zD.*zI.*2.0;
t699 = yD.*yJ.*zI.*zJ.*2.0;
t700 = yI.*yJ.*zD.*zJ.*2.0;
t844 = t13.*xD.*xI.*2.0;
t845 = t5.*xD.*xJ.*2.0;
t846 = t4.*xI.*xJ.*2.0;
t847 = t15.*xD.*xI.*2.0;
t848 = t7.*xD.*xJ.*2.0;
t849 = t6.*xI.*xJ.*2.0;
t850 = t2.*yI.*yJ.*2.0;
t851 = t3.*yD.*yJ.*2.0;
t852 = t14.*yD.*yI.*2.0;
t853 = t15.*yD.*yI.*2.0;
t854 = t7.*yD.*yJ.*2.0;
t855 = t6.*yI.*yJ.*2.0;
t856 = t2.*zI.*zJ.*2.0;
t857 = t3.*zD.*zJ.*2.0;
t858 = t14.*zD.*zI.*2.0;
t859 = t4.*zI.*zJ.*2.0;
t860 = t5.*zD.*zJ.*2.0;
t861 = t13.*zD.*zI.*2.0;
t862 = xD.*xI.*yD.*yI.*2.0;
t863 = xD.*xJ.*yD.*yJ.*2.0;
t864 = xI.*xJ.*yI.*yJ.*2.0;
t865 = xD.*xI.*zD.*zI.*2.0;
t866 = xD.*xJ.*zD.*zJ.*2.0;
t867 = xI.*xJ.*zI.*zJ.*2.0;
t868 = yD.*yI.*zD.*zI.*2.0;
t869 = yD.*yJ.*zD.*zJ.*2.0;
t870 = yI.*yJ.*zI.*zJ.*2.0;
t701 = t665+t666+t667+t668+t669+t670+t671+t672+t673+t674+t675+t676+t677+t678+t679+t680+t681+t682+t683+t684+t685+t686+t687+t688+t689+t690+t691+t692+t693+t694+t695+t696+t697+t698+t699+t700-t844-t845-t846-t847-t848-t849-t850-t851-t852-t853-t854-t855-t856-t857-t858-t859-t860-t861-t862-t863-t864-t865-t866-t867-t868-t869-t870;
t702 = 1.0./t701;
t703 = t2.*t7.*zI.*2.0;
t704 = t3.*t6.*zD;
t705 = t6.*t14.*zD;
t706 = t7.*t14.*zI;
t707 = t4.*t7.*zI.*2.0;
t708 = t5.*t6.*zD;
t709 = t6.*t13.*zD;
t710 = t7.*t13.*zI;
t711 = t16.*zD;
t712 = t3.*zJ.*3.729e3;
t713 = t14.*zI.*3.729e3;
t714 = t17.*zD;
t715 = t5.*zJ.*3.729e3;
t716 = t13.*zI.*3.729e3;
t717 = t3.*xD.*xI.*zJ.*3.0;
t718 = t2.*xD.*xI.*zJ;
t719 = t2.*xD.*xJ.*zI;
t720 = t7.*xI.*xJ.*zI;
t721 = t3.*xI.*xJ.*zI;
t722 = t3.*xI.*xJ.*zJ;
t723 = t5.*yD.*yI.*zJ.*3.0;
t724 = t4.*yD.*yI.*zJ;
t725 = t4.*yD.*yJ.*zI;
t726 = t7.*yI.*yJ.*zI;
t727 = t5.*yI.*yJ.*zI;
t728 = t5.*yI.*yJ.*zJ;
t729 = t2.*t3.*zD;
t730 = t2.*t14.*zD;
t731 = t2.*t3.*zI.*2.0;
t732 = t3.*t14.*zD;
t733 = t2.*t5.*zD;
t734 = t3.*t4.*zD;
t735 = t2.*t13.*zD;
t736 = t4.*t14.*zD;
t737 = t2.*t5.*zI.*2.0;
t738 = t3.*t4.*zI.*2.0;
t739 = t3.*t5.*zD.*2.0;
t740 = t2.*t13.*zI;
t741 = t3.*t13.*zD;
t742 = t4.*t14.*zI;
t743 = t5.*t14.*zD;
t744 = t3.*t13.*zI;
t745 = t5.*t14.*zI;
t746 = t4.*t5.*zD;
t747 = t4.*t13.*zD;
t748 = t3.*t7.*zD;
t749 = t4.*t5.*zI.*2.0;
t750 = t2.*t15.*zI.*2.0;
t751 = t5.*t13.*zD;
t752 = t3.*t15.*zI.*2.0;
t753 = t5.*t7.*zD;
t754 = t4.*t15.*zI.*2.0;
t755 = t5.*t15.*zI.*2.0;
t756 = t2.*t5.*t476.*2.0;
t757 = t3.*t4.*t476.*2.0;
t758 = t2.*t13.*t476.*2.0;
t759 = t4.*t14.*t476.*2.0;
t760 = t3.*t13.*t476.*2.0;
t761 = t5.*t14.*t476.*2.0;
t762 = t2.*t7.*t476.*2.0;
t763 = t3.*t6.*t476.*2.0;
t764 = t2.*t15.*t476.*2.0;
t765 = t6.*t14.*t476.*2.0;
t766 = t3.*t15.*t476.*2.0;
t767 = t7.*t14.*t476.*2.0;
t768 = t4.*t7.*t476.*2.0;
t769 = t5.*t6.*t476.*2.0;
t770 = t4.*t15.*t476.*2.0;
t771 = t6.*t13.*t476.*2.0;
t772 = t5.*t15.*t476.*2.0;
t773 = t7.*t13.*t476.*2.0;
t774 = xD.*xI.*zI.*3.729e3;
t775 = xI.*xJ.*zD.*7.458e3;
t776 = xD.*xJ.*zJ.*3.729e3;
t777 = yD.*yI.*zI.*3.729e3;
t778 = yI.*yJ.*zD.*7.458e3;
t779 = yD.*yJ.*zJ.*3.729e3;
t780 = t3.*xD.*xJ.*zD.*4.0;
t781 = t14.*xD.*xI.*zI.*2.0;
t782 = t2.*xI.*xJ.*zJ.*3.0;
t783 = t4.*xD.*xI.*zJ;
t784 = t4.*xD.*xJ.*zI;
t785 = t5.*xD.*xI.*zJ.*3.0;
t786 = t4.*xI.*xJ.*zJ;
t787 = t5.*xI.*xJ.*zI;
t788 = t5.*xI.*xJ.*zJ;
t789 = t6.*xD.*xI.*zJ;
t790 = t7.*xD.*xJ.*zD.*2.0;
t791 = t6.*xD.*xJ.*zI;
t792 = t2.*yD.*yI.*zJ;
t793 = t2.*yD.*yJ.*zI;
t794 = t7.*xD.*xI.*zJ.*5.0;
t795 = t6.*xI.*xJ.*zI;
t796 = t3.*yD.*yI.*zJ.*3.0;
t797 = t7.*xD.*xJ.*zJ.*3.0;
t798 = t6.*xI.*xJ.*zJ;
t799 = t2.*yI.*yJ.*zJ;
t800 = t3.*yI.*yJ.*zI;
t801 = t3.*yI.*yJ.*zJ;
t802 = t5.*yD.*yJ.*zD.*4.0;
t803 = t13.*yD.*yI.*zI.*2.0;
t804 = t4.*yI.*yJ.*zJ.*3.0;
t805 = t6.*yD.*yI.*zJ;
t806 = t7.*yD.*yJ.*zD.*2.0;
t807 = t6.*yD.*yJ.*zI;
t808 = t7.*yD.*yI.*zJ.*5.0;
t809 = t6.*yI.*yJ.*zI;
t810 = t7.*yD.*yJ.*zJ.*3.0;
t811 = t6.*yI.*yJ.*zJ;
t812 = xD.*xI.*yD.*yJ.*zI.*2.0;
t813 = xD.*xI.*yI.*yJ.*zD.*4.0;
t814 = xD.*xJ.*yD.*yI.*zI.*2.0;
t815 = xI.*xJ.*yD.*yI.*zD.*4.0;
t816 = xD.*xI.*yD.*yJ.*zJ.*2.0;
t817 = xD.*xJ.*yD.*yI.*zJ.*2.0;
t818 = xD.*xI.*yI.*yJ.*zI.*2.0;
t819 = xI.*xJ.*yD.*yI.*zI.*2.0;
t820 = xD.*xJ.*yI.*yJ.*zI.*4.0;
t821 = xI.*xJ.*yD.*yJ.*zI.*4.0;
t822 = xD.*xI.*zD.*zI.*zJ.*2.0;
t823 = xI.*xJ.*zD.*zI.*zJ.*2.0;
t824 = yD.*yI.*zD.*zI.*zJ.*2.0;
t825 = yI.*yJ.*zD.*zI.*zJ.*2.0;
t826 = t476.*xD.*xI.*yD.*yJ.*4.0;
t827 = t476.*xD.*xJ.*yD.*yI.*4.0;
t828 = t476.*xD.*xI.*yI.*yJ.*4.0;
t829 = t476.*xI.*xJ.*yD.*yI.*4.0;
t830 = t476.*xD.*xJ.*yI.*yJ.*4.0;
t831 = t476.*xI.*xJ.*yD.*yJ.*4.0;
t832 = t476.*xD.*xI.*zD.*zJ.*4.0;
t833 = t476.*xD.*xJ.*zD.*zI.*4.0;
t834 = t476.*xD.*xI.*zI.*zJ.*4.0;
t835 = t476.*xI.*xJ.*zD.*zI.*4.0;
t836 = t476.*xD.*xJ.*zI.*zJ.*4.0;
t837 = t476.*xI.*xJ.*zD.*zJ.*4.0;
t838 = t476.*yD.*yI.*zD.*zJ.*4.0;
t839 = t476.*yD.*yJ.*zD.*zI.*4.0;
t840 = t476.*yD.*yI.*zI.*zJ.*4.0;
t841 = t476.*yI.*yJ.*zD.*zI.*4.0;
t842 = t476.*yD.*yJ.*zI.*zJ.*4.0;
t843 = t476.*yI.*yJ.*zD.*zJ.*4.0;
t871 = t3.*zD.*3.729e3;
t872 = t14.*zD.*3.729e3;
t873 = t16.*zJ;
t874 = t5.*zD.*3.729e3;
t875 = t13.*zD.*3.729e3;
t876 = t17.*zJ;
t877 = t3.*xD.*xI.*zD.*2.0;
t878 = t7.*xD.*xI.*zI;
t879 = t3.*xD.*xI.*zI;
t880 = t2.*xD.*xI.*zI;
t881 = t7.*xD.*xJ.*zI.*3.0;
t882 = t6.*xI.*xJ.*zD.*2.0;
t883 = t3.*xI.*xJ.*zD.*2.0;
t884 = t2.*xD.*xJ.*zJ;
t885 = t5.*yD.*yI.*zD.*2.0;
t886 = t7.*yD.*yI.*zI;
t887 = t5.*yD.*yI.*zI;
t888 = t4.*yD.*yI.*zI;
t889 = t7.*yD.*yJ.*zI.*3.0;
t890 = t6.*yI.*yJ.*zD.*2.0;
t891 = t5.*yI.*yJ.*zD.*2.0;
t892 = t4.*yD.*yJ.*zJ;
t893 = t2.*t3.*zJ.*3.0;
t894 = t2.*t14.*zI;
t895 = t3.*t14.*zI;
t896 = t2.*t5.*zJ;
t897 = t3.*t4.*zJ;
t898 = t3.*t5.*zJ.*2.0;
t899 = t2.*t7.*zJ.*4.0;
t900 = t3.*t6.*zJ;
t901 = t7.*t14.*zD;
t902 = t6.*t14.*zI;
t903 = t4.*t5.*zJ.*3.0;
t904 = t4.*t13.*zI;
t905 = t3.*t7.*zJ;
t906 = t5.*t13.*zI;
t907 = t4.*t7.*zJ.*4.0;
t908 = t5.*t6.*zJ;
t909 = t7.*t13.*zD;
t910 = t6.*t13.*zI;
t911 = t5.*t7.*zJ;
t912 = xD.*xI.*zJ.*3.729e3;
t913 = xD.*xJ.*zI.*3.729e3;
t914 = xI.*xJ.*zI.*3.729e3;
t915 = xI.*xJ.*zJ.*3.729e3;
t916 = yD.*yI.*zJ.*3.729e3;
t917 = yD.*yJ.*zI.*3.729e3;
t918 = yI.*yJ.*zI.*3.729e3;
t919 = yI.*yJ.*zJ.*3.729e3;
t920 = t14.*xD.*xI.*zD.*2.0;
t921 = t2.*xI.*xJ.*zD.*2.0;
t922 = t3.*xD.*xJ.*zI;
t923 = t2.*xI.*xJ.*zI;
t924 = t3.*xD.*xJ.*zJ.*3.0;
t925 = t4.*xD.*xI.*zI;
t926 = t5.*xD.*xI.*zD.*2.0;
t927 = t13.*xD.*xI.*zD.*2.0;
t928 = t4.*xI.*xJ.*zD.*2.0;
t929 = t4.*xD.*xJ.*zJ;
t930 = t5.*xD.*xI.*zI;
t931 = t13.*xD.*xI.*zI.*2.0;
t932 = t5.*xD.*xJ.*zI.*3.0;
t933 = t4.*xI.*xJ.*zI.*3.0;
t934 = t5.*xI.*xJ.*zD.*2.0;
t935 = t5.*xD.*xJ.*zJ;
t936 = t7.*xD.*xI.*zD.*2.0;
t937 = t6.*xD.*xI.*zI;
t938 = t2.*yD.*yI.*zI;
t939 = t3.*yD.*yI.*zD.*2.0;
t940 = t2.*yI.*yJ.*zD.*2.0;
t941 = t14.*yD.*yI.*zD.*2.0;
t942 = t6.*xD.*xJ.*zJ;
t943 = t2.*yD.*yJ.*zJ;
t944 = t3.*yD.*yI.*zI;
t945 = t15.*xD.*xI.*zI.*4.0;
t946 = t2.*yI.*yJ.*zI.*3.0;
t947 = t3.*yD.*yJ.*zI.*3.0;
t948 = t3.*yI.*yJ.*zD.*2.0;
t949 = t14.*yD.*yI.*zI.*2.0;
t950 = t3.*yD.*yJ.*zJ;
t951 = t7.*xI.*xJ.*zJ.*3.0;
t952 = t13.*yD.*yI.*zD.*2.0;
t953 = t4.*yI.*yJ.*zD.*2.0;
t954 = t5.*yD.*yJ.*zI;
t955 = t4.*yI.*yJ.*zI;
t956 = t5.*yD.*yJ.*zJ.*3.0;
t957 = t7.*yD.*yI.*zD.*2.0;
t958 = t6.*yD.*yI.*zI;
t959 = t6.*yD.*yJ.*zJ;
t960 = t15.*yD.*yI.*zI.*4.0;
t961 = t3.*zD.*zI.*zJ.*2.0;
t962 = t7.*yI.*yJ.*zJ.*3.0;
t963 = t5.*zD.*zI.*zJ.*2.0;
t964 = xD.*xI.*yD.*yI.*zJ.*4.0;
t965 = xD.*xJ.*yD.*yJ.*zI.*4.0;
t966 = xD.*xI.*yI.*yJ.*zJ.*2.0;
t967 = xI.*xJ.*yD.*yI.*zJ.*2.0;
t968 = xI.*xJ.*yI.*yJ.*zI.*4.0;
t969 = xD.*xJ.*zD.*zI.*zJ.*2.0;
t970 = yD.*yJ.*zD.*zI.*zJ.*2.0;
t971 = xJ.*3.729e3;
t972 = t2.*xI;
t973 = t4.*xI;
t974 = t5.*xI;
t975 = t5.*xJ;
t976 = t6.*xI;
t977 = t7.*xI;
t978 = t7.*xJ;
t979 = xD.*xI.*xJ.*2.0;
t980 = xD.*yI.*yJ.*2.0;
t981 = xD.*zI.*zJ.*2.0;
t982 = t971+t972+t973+t974+t975+t976+t977+t978+t979+t980+t981-xI.*3.729e3-t3.*xD.*2.0-t5.*xD.*2.0-t7.*xD.*2.0+t3.*xI-t2.*xJ-t3.*xJ-t4.*xJ-t6.*xJ-xI.*yI.*yJ.*2.0-xI.*zI.*zJ.*2.0;
t983 = xD.*zI;
t984 = xJ.*zD;
t985 = xI.*zJ;
t986 = t983+t984+t985-xI.*zD-xD.*zJ-xJ.*zI;
t988 = t13.*t476.*xD.*xI.*4.0;
t989 = t5.*t476.*xD.*xJ.*4.0;
t990 = t4.*t476.*xI.*xJ.*4.0;
t991 = t15.*t476.*xD.*xI.*4.0;
t992 = t7.*t476.*xD.*xJ.*4.0;
t993 = t6.*t476.*xI.*xJ.*4.0;
t994 = t2.*t476.*yI.*yJ.*4.0;
t995 = t3.*t476.*yD.*yJ.*4.0;
t996 = t14.*t476.*yD.*yI.*4.0;
t997 = t15.*t476.*yD.*yI.*4.0;
t998 = t7.*t476.*yD.*yJ.*4.0;
t999 = t6.*t476.*yI.*yJ.*4.0;
t1000 = t2.*t476.*zI.*zJ.*4.0;
t1001 = t3.*t476.*zD.*zJ.*4.0;
t1002 = t14.*t476.*zD.*zI.*4.0;
t1003 = t4.*t476.*zI.*zJ.*4.0;
t1004 = t5.*t476.*zD.*zJ.*4.0;
t1005 = t13.*t476.*zD.*zI.*4.0;
t1006 = t476.*xD.*xI.*yD.*yI.*4.0;
t1007 = t476.*xD.*xJ.*yD.*yJ.*4.0;
t1008 = t476.*xI.*xJ.*yI.*yJ.*4.0;
t1009 = t476.*xD.*xI.*zD.*zI.*4.0;
t1010 = t476.*xD.*xJ.*zD.*zJ.*4.0;
t1011 = t476.*xI.*xJ.*zI.*zJ.*4.0;
t1012 = t476.*yD.*yI.*zD.*zI.*4.0;
t1013 = t476.*yD.*yJ.*zD.*zJ.*4.0;
t1014 = t476.*yI.*yJ.*zI.*zJ.*4.0;
t987 = -t703-t704-t705-t706-t707-t708-t709-t710-t711-t712-t713-t714-t715-t716-t717-t718-t719-t720-t721-t722-t723-t724-t725-t726-t727-t728-t729-t730-t731-t732-t733-t734-t735-t736-t737-t738-t739-t740-t741-t742-t743-t744-t745-t746-t747-t748-t749-t750-t751-t752-t753-t754-t755+t756+t757+t758+t759+t760+t761+t762+t763+t764+t765+t766+t767+t768+t769+t770+t771+t772+t773-t774-t775-t776-t777-t778-t779-t780-t781-t782-t783-t784-t785-t786-t787-t788-t789-t790-t791-t792-t793-t794-t795-t796-t797-t798-t799-t800-t801-t802-t803-t804-t805-t806-t807-t808-t809-t810-t811-t812-t813-t814-t815-t816-t817-t818-t819-t820-t821-t822-t823-t824-t825+t826+t827+t828+t829+t830+t831+t832+t833+t834+t835+t836+t837+t838+t839+t840+t841+t842+t843+t871+t872+t873+t874+t875+t876+t877+t878+t879+t880+t881+t882+t883+t884+t885+t886+t887+t888+t889+t890+t891+t892+t893+t894+t895+t896+t897+t898+t899+t900+t901+t902+t903+t904+t905+t906+t907+t908+t909+t910+t911+t912+t913+t914+t915+t916+t917+t918+t919+t920+t921+t922+t923+t924+t925+t926+t927+t928+t929+t930+t931+t932+t933+t934+t935+t936+t937+t938+t939+t940+t941+t942+t943+t944+t945+t946+t947+t948+t949+t950+t951+t952+t953+t954+t955+t956+t957+t958+t959+t960+t961+t962+t963+t964+t965+t966+t967+t968+t969+t970-t988-t989-t990-t991-t992-t993-t994-t995-t996-t997-t998-t999-t1000-t1001-t1002-t1003-t1004-t1005-t1006-t1007-t1008-t1009-t1010-t1011-t1012-t1013-t1014;
xH_sol = [t660+t12.*t664.*t702.*(t703+t704+t705+t706+t707+t708+t709+t710+t711+t712+t713+t714+t715+t716+t717+t718+t719+t720+t721+t722+t723+t724+t725+t726+t727+t728+t729+t730+t731+t732+t733+t734+t735+t736+t737+t738+t739+t740+t741+t742+t743+t744+t745+t746+t747+t748+t749+t750+t751+t752+t753+t754+t755+t756+t757+t758+t759+t760+t761+t762+t763+t764+t765+t766+t767+t768+t769+t770+t771+t772+t773+t774+t775+t776+t777+t778+t779+t780+t781+t782+t783+t784+t785+t786+t787+t788+t789+t790+t791+t792+t793+t794+t795+t796+t797+t798+t799+t800+t801+t802+t803+t804+t805+t806+t807+t808+t809+t810+t811+t812+t813+t814+t815+t816+t817+t818+t819+t820+t821+t822+t823+t824+t825+t826+t827+t828+t829+t830+t831+t832+t833+t834+t835+t836+t837+t838+t839+t840+t841+t842+t843-t3.*zD.*3.729e3-t5.*zD.*3.729e3-t13.*zD.*3.729e3-t14.*zD.*3.729e3-t16.*zJ-t17.*zJ-t7.*t13.*zD-t7.*t14.*zD-t2.*t14.*zI-t3.*t14.*zI-t4.*t13.*zI-t5.*t13.*zI-t6.*t13.*zI-t6.*t14.*zI-t2.*t3.*zJ.*3.0-t2.*t5.*zJ-t3.*t4.*zJ-t3.*t5.*zJ.*2.0-t2.*t7.*zJ.*4.0-t3.*t6.*zJ-t4.*t5.*zJ.*3.0-t3.*t7.*zJ-t4.*t7.*zJ.*4.0-t5.*t6.*zJ-t5.*t7.*zJ-xD.*xI.*zJ.*3.729e3-xD.*xJ.*zI.*3.729e3-xI.*xJ.*zI.*3.729e3-xI.*xJ.*zJ.*3.729e3-yD.*yI.*zJ.*3.729e3-yD.*yJ.*zI.*3.729e3-yI.*yJ.*zI.*3.729e3-yI.*yJ.*zJ.*3.729e3-t13.*t476.*xD.*xI.*4.0-t15.*t476.*xD.*xI.*4.0-t5.*t476.*xD.*xJ.*4.0-t7.*t476.*xD.*xJ.*4.0-t4.*t476.*xI.*xJ.*4.0-t6.*t476.*xI.*xJ.*4.0-t14.*t476.*yD.*yI.*4.0-t15.*t476.*yD.*yI.*4.0-t3.*t476.*yD.*yJ.*4.0-t7.*t476.*yD.*yJ.*4.0-t2.*t476.*yI.*yJ.*4.0-t6.*t476.*yI.*yJ.*4.0-t13.*t476.*zD.*zI.*4.0-t14.*t476.*zD.*zI.*4.0-t3.*t476.*zD.*zJ.*4.0-t5.*t476.*zD.*zJ.*4.0-t2.*t476.*zI.*zJ.*4.0-t4.*t476.*zI.*zJ.*4.0-t3.*xD.*xI.*zD.*2.0-t5.*xD.*xI.*zD.*2.0-t7.*xD.*xI.*zD.*2.0-t13.*xD.*xI.*zD.*2.0-t14.*xD.*xI.*zD.*2.0-t2.*xD.*xI.*zI-t3.*xD.*xI.*zI-t4.*xD.*xI.*zI-t5.*xD.*xI.*zI-t6.*xD.*xI.*zI-t7.*xD.*xI.*zI-t13.*xD.*xI.*zI.*2.0-t15.*xD.*xI.*zI.*4.0-t2.*xI.*xJ.*zD.*2.0-t3.*xD.*xJ.*zI-t3.*xI.*xJ.*zD.*2.0-t4.*xI.*xJ.*zD.*2.0-t5.*xD.*xJ.*zI.*3.0-t5.*xI.*xJ.*zD.*2.0-t6.*xI.*xJ.*zD.*2.0-t7.*xD.*xJ.*zI.*3.0-t2.*xD.*xJ.*zJ-t3.*xD.*xJ.*zJ.*3.0-t4.*xD.*xJ.*zJ-t5.*xD.*xJ.*zJ-t6.*xD.*xJ.*zJ-t2.*xI.*xJ.*zI-t4.*xI.*xJ.*zI.*3.0-t7.*xI.*xJ.*zJ.*3.0-t3.*yD.*yI.*zD.*2.0-t5.*yD.*yI.*zD.*2.0-t7.*yD.*yI.*zD.*2.0-t13.*yD.*yI.*zD.*2.0-t14.*yD.*yI.*zD.*2.0-t2.*yD.*yI.*zI-t3.*yD.*yI.*zI-t4.*yD.*yI.*zI-t5.*yD.*yI.*zI-t6.*yD.*yI.*zI-t7.*yD.*yI.*zI-t14.*yD.*yI.*zI.*2.0-t15.*yD.*yI.*zI.*4.0-t2.*yI.*yJ.*zD.*2.0-t3.*yD.*yJ.*zI.*3.0-t3.*yI.*yJ.*zD.*2.0-t4.*yI.*yJ.*zD.*2.0-t5.*yD.*yJ.*zI-t5.*yI.*yJ.*zD.*2.0-t6.*yI.*yJ.*zD.*2.0-t7.*yD.*yJ.*zI.*3.0-t2.*yD.*yJ.*zJ-t3.*yD.*yJ.*zJ-t4.*yD.*yJ.*zJ-t5.*yD.*yJ.*zJ.*3.0-t6.*yD.*yJ.*zJ-t2.*yI.*yJ.*zI.*3.0-t4.*yI.*yJ.*zI-t7.*yI.*yJ.*zJ.*3.0-t3.*zD.*zI.*zJ.*2.0-t5.*zD.*zI.*zJ.*2.0-t476.*xD.*xI.*yD.*yI.*4.0-t476.*xD.*xJ.*yD.*yJ.*4.0-t476.*xI.*xJ.*yI.*yJ.*4.0-t476.*xD.*xI.*zD.*zI.*4.0-t476.*xD.*xJ.*zD.*zJ.*4.0-t476.*xI.*xJ.*zI.*zJ.*4.0-t476.*yD.*yI.*zD.*zI.*4.0-t476.*yD.*yJ.*zD.*zJ.*4.0-t476.*yI.*yJ.*zI.*zJ.*4.0-xD.*xI.*yD.*yI.*zJ.*4.0-xD.*xJ.*yD.*yJ.*zI.*4.0-xD.*xI.*yI.*yJ.*zJ.*2.0-xI.*xJ.*yD.*yI.*zJ.*2.0-xI.*xJ.*yI.*yJ.*zI.*4.0-xD.*xJ.*zD.*zI.*zJ.*2.0-yD.*yJ.*zD.*zI.*zJ.*2.0).*(1.0./2.0);t660-t12.*t664.*t702.*t987.*(1.0./2.0)];
if nargout > 1
    yH_sol = [t12.*t982.*(-1.0./2.0)-t12.*t702.*t986.*(t703+t704+t705+t706+t707+t708+t709+t710+t711+t712+t713+t714+t715+t716+t717+t718+t719+t720+t721+t722+t723+t724+t725+t726+t727+t728+t729+t730+t731+t732+t733+t734+t735+t736+t737+t738+t739+t740+t741+t742+t743+t744+t745+t746+t747+t748+t749+t750+t751+t752+t753+t754+t755+t756+t757+t758+t759+t760+t761+t762+t763+t764+t765+t766+t767+t768+t769+t770+t771+t772+t773+t774+t775+t776+t777+t778+t779+t780+t781+t782+t783+t784+t785+t786+t787+t788+t789+t790+t791+t792+t793+t794+t795+t796+t797+t798+t799+t800+t801+t802+t803+t804+t805+t806+t807+t808+t809+t810+t811+t812+t813+t814+t815+t816+t817+t818+t819+t820+t821+t822+t823+t824+t825+t826+t827+t828+t829+t830+t831+t832+t833+t834+t835+t836+t837+t838+t839+t840+t841+t842+t843-t871-t872-t873-t874-t875-t876-t877-t878-t879-t880-t881-t882-t883-t884-t885-t886-t887-t888-t889-t890-t891-t892-t893-t894-t895-t896-t897-t898-t899-t900-t901-t902-t903-t904-t905-t906-t907-t908-t909-t910-t911-t912-t913-t914-t915-t916-t917-t918-t919-t920-t921-t922-t923-t924-t925-t926-t927-t928-t929-t930-t931-t932-t933-t934-t935-t936-t937-t938-t939-t940-t941-t942-t943-t944-t945-t946-t947-t948-t949-t950-t951-t952-t953-t954-t955-t956-t957-t958-t959-t960-t961-t962-t963-t964-t965-t966-t967-t968-t969-t970-t13.*t476.*xD.*xI.*4.0-t15.*t476.*xD.*xI.*4.0-t5.*t476.*xD.*xJ.*4.0-t7.*t476.*xD.*xJ.*4.0-t4.*t476.*xI.*xJ.*4.0-t6.*t476.*xI.*xJ.*4.0-t14.*t476.*yD.*yI.*4.0-t15.*t476.*yD.*yI.*4.0-t3.*t476.*yD.*yJ.*4.0-t7.*t476.*yD.*yJ.*4.0-t2.*t476.*yI.*yJ.*4.0-t6.*t476.*yI.*yJ.*4.0-t13.*t476.*zD.*zI.*4.0-t14.*t476.*zD.*zI.*4.0-t3.*t476.*zD.*zJ.*4.0-t5.*t476.*zD.*zJ.*4.0-t2.*t476.*zI.*zJ.*4.0-t4.*t476.*zI.*zJ.*4.0-t476.*xD.*xI.*yD.*yI.*4.0-t476.*xD.*xJ.*yD.*yJ.*4.0-t476.*xI.*xJ.*yI.*yJ.*4.0-t476.*xD.*xI.*zD.*zI.*4.0-t476.*xD.*xJ.*zD.*zJ.*4.0-t476.*xI.*xJ.*zI.*zJ.*4.0-t476.*yD.*yI.*zD.*zI.*4.0-t476.*yD.*yJ.*zD.*zJ.*4.0-t476.*yI.*yJ.*zI.*zJ.*4.0).*(1.0./2.0);t12.*t982.*(-1.0./2.0)+t12.*t702.*t986.*t987.*(1.0./2.0)];
end
if nargout > 2
    zH_sol = [t702.*(t703+t704+t705+t706+t707+t708+t709+t710+t711+t712+t713+t714+t715+t716+t717+t718+t719+t720+t721+t722+t723+t724+t725+t726+t727+t728+t729+t730+t731+t732+t733+t734+t735+t736+t737+t738+t739+t740+t741+t742+t743+t744+t745+t746+t747+t748+t749+t750+t751+t752+t753+t754+t755+t756+t757+t758+t759+t760+t761+t762+t763+t764+t765+t766+t767+t768+t769+t770+t771+t772+t773+t774+t775+t776+t777+t778+t779+t780+t781+t782+t783+t784+t785+t786+t787+t788+t789+t790+t791+t792+t793+t794+t795+t796+t797+t798+t799+t800+t801+t802+t803+t804+t805+t806+t807+t808+t809+t810+t811+t812+t813+t814+t815+t816+t817+t818+t819+t820+t821+t822+t823+t824+t825+t826+t827+t828+t829+t830+t831+t832+t833+t834+t835+t836+t837+t838+t839+t840+t841+t842+t843-t871-t872-t873-t874-t875-t876-t877-t878-t879-t880-t881-t882-t883-t884-t885-t886-t887-t888-t889-t890-t891-t892-t893-t894-t895-t896-t897-t898-t899-t900-t901-t902-t903-t904-t905-t906-t907-t908-t909-t910-t911-t912-t913-t914-t915-t916-t917-t918-t919-t920-t921-t922-t923-t924-t925-t926-t927-t928-t929-t930-t931-t932-t933-t934-t935-t936-t937-t938-t939-t940-t941-t942-t943-t944-t945-t946-t947-t948-t949-t950-t951-t952-t953-t954-t955-t956-t957-t958-t959-t960-t961-t962-t963-t964-t965-t966-t967-t968-t969-t970-t988-t989-t990-t991-t992-t993-t994-t995-t996-t997-t998-t999-t1000-t1001-t1002-t1003-t1004-t1005-t1006-t1007-t1008-t1009-t1010-t1011-t1012-t1013-t1014).*(1.0./2.0);t702.*t987.*(-1.0./2.0)];
end
end

== matlab function dx_hand_model/Thumb/Direct Kinematics/get H/MATLAB Function4 ==
  data: u input; d output
function d = fcn(u)

d = sqrt(u(1)^2+u(2)^2+u(3)^2);
